simulink subsystem "Voltage_to_duty_1"  (R2024a)
settings: Solver=VariableStepAuto  StartTime=0.0  StopTime=10.0  RelTol=1e-3
settings Model: Creator=Peter  LastModifiedBy=Peter

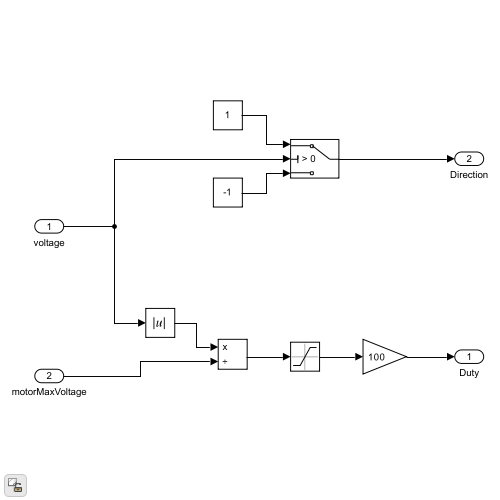
[thumbnail: Simulink's stored preview of the top-level diagram]
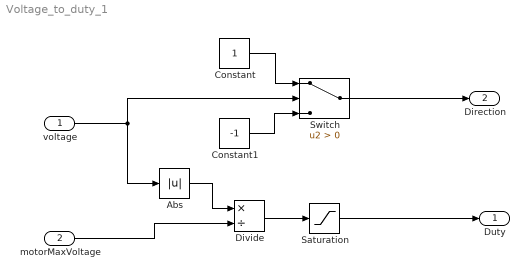
== system Voltage_to_duty_1 ==
  voltage : Inport  OutDataTypeStr=single
  motorMaxVoltage : Inport  Port=2  OutDataTypeStr=single
  Abs : Abs  SaturateOnIntegerOverflow=off
  Constant : Constant  OutDataTypeStr=int8
  Constant1 : Constant  Value=-1  OutDataTypeStr=int8
  Divide : Product  Inputs=*/
  Saturation : Saturate  UpperLimit=1  LowerLimit=0
  Switch : Switch  Criteria=u2 > Threshold  OutDataTypeStr=int8  SaturateOnIntegerOverflow=off  InputSameDT=off
  Duty : Outport  OutDataTypeStr=single
  Direction : Outport  Port=2  OutDataTypeStr=int8
  wires:
  Constant/1 -> Switch/1
  motorMaxVoltage/1 -> Divide/2
  Switch/1 -> Direction/1
  Constant1/1 -> Switch/3
  Divide/1 -> Saturation/1
  voltage/1 -> Abs/1, Switch/2
  Abs/1 -> Divide/1
  Saturation/1 -> Duty/1
